simulink model "position_integrator"  (R2023b)
settings: Solver=ode15s  StartTime=0.0  StopTime=1  RelTol=1e-10
undefined symbols (not defined in the file): K, Ki
settings Model: PacingRate=1000  Creator=franc  LastModifiedBy=Beniamino

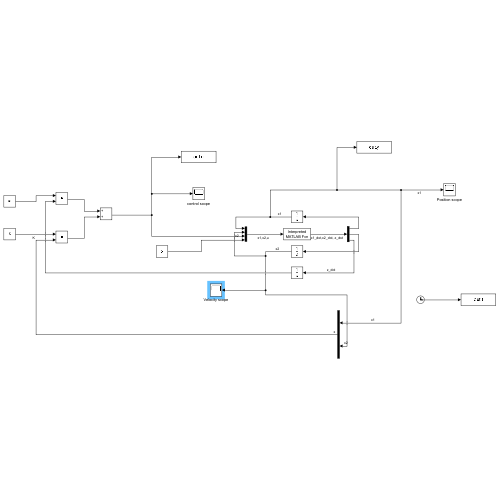
[thumbnail: Simulink's stored preview of the top-level diagram]
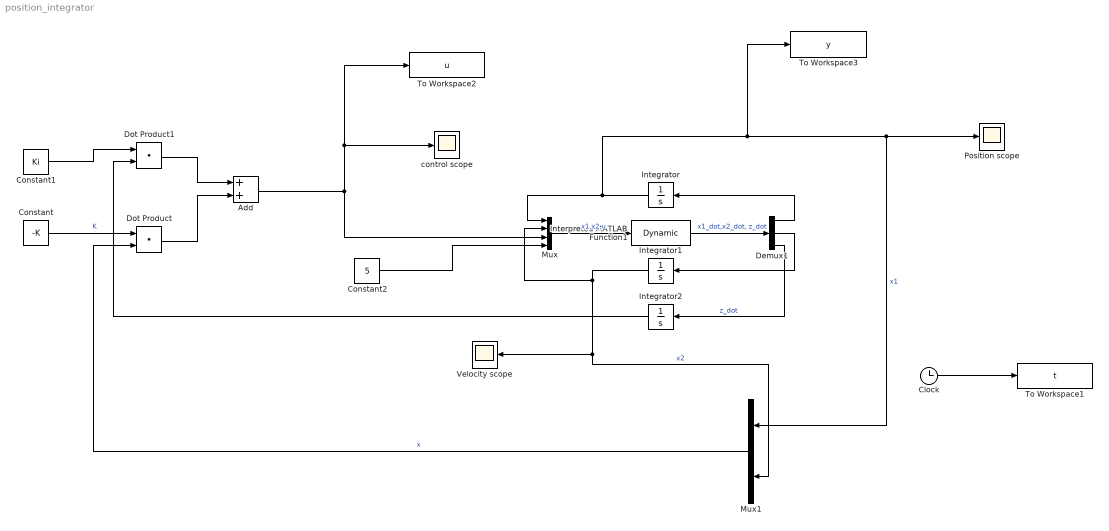
== system position_integrator ==
  Add : Sum
  Clock : Clock
  Constant : Constant  Value=-K
  Constant1 : Constant  Value=Ki
  Constant2 : Constant  Value=5
  Demux1 : Demux  Outputs=3
  Dot Product : DotProduct  OutDataTypeStr=Inherit: Inherit via internal rule
  Dot Product1 : DotProduct  OutDataTypeStr=Inherit: Inherit via internal rule
  Integrator : Integrator
  Integrator1 : Integrator
  Integrator2 : Integrator
  Interpreted MATLAB Function1 : MATLABFcn  MATLABFcn=Dynamic  OutputDimensions=3
  Mux : Mux
  Mux1 : Mux  Inputs=2
  Position scope : Scope
  To Workspace1 : ToWorkspace  VariableName=t  SampleTime=-1
  To Workspace2 : ToWorkspace  VariableName=u  SampleTime=-1
  To Workspace3 : ToWorkspace  VariableName=y  SampleTime=-1
  Velocity scope : Scope
  control scope : Scope
  wires:
  Interpreted MATLAB Function1/1 -> Demux1/1  "x1_dot,x2_dot, z_dot"
  Constant/1 -> Dot Product/1  "K"
  Demux1/2 -> Integrator1/1
  Demux1/1 -> Integrator/1
  Mux/1 -> Interpreted MATLAB Function1/1  "x1,x2,u"
  Integrator/1 -> To Workspace3/1, Mux1/1, Position scope/1, Mux/1  "x1"
  Integrator1/1 -> Mux1/2, Velocity scope/1, Mux/2  "x2"
  Clock/1 -> To Workspace1/1
  Mux1/1 -> Dot Product/2  "x"
  Demux1/3 -> Integrator2/1  "z_dot"
  Constant1/1 -> Dot Product1/1
  Integrator2/1 -> Dot Product1/2
  Dot Product1/1 -> Add/1
  Dot Product/1 -> Add/2
  Add/1 -> To Workspace2/1, control scope/1, Mux/3
  Constant2/1 -> Mux/4
